simulink model "pendule_simple"  (R2023a)
settings: Solver=VariableStepAuto  StartTime=0.0  StopTime=10.0  RelTol=1e-3
undefined symbols (not defined in the file): g, l
settings Model: Creator=pmt1554  LastModifiedBy=pmt1554

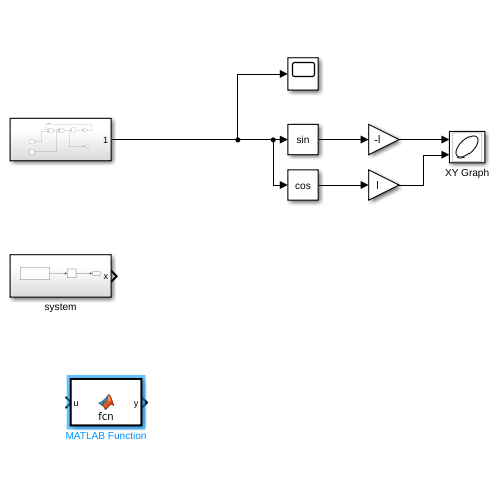
[thumbnail: Simulink's stored preview of the top-level diagram]
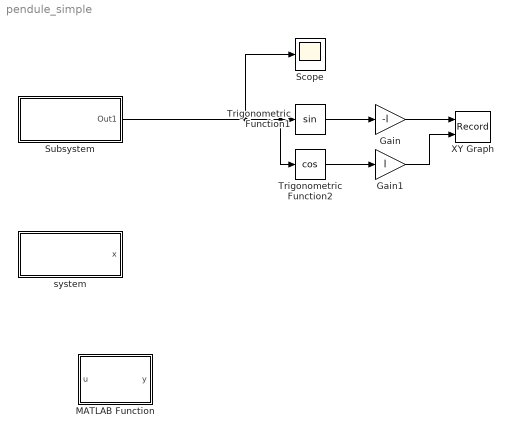
== system pendule_simple ==
  Gain : Gain  Gain=-l
  Gain1 : Gain  Gain=l
  MATLAB Function : MATLAB Function  TreatAsAtomicUnit=on
  Scope : Scope
  Subsystem : Subsystem
  Trigonometric Function1 : Trigonometry
  Trigonometric Function2 : Trigonometry  Operator=cos
  XY Graph : Record  FileSettingsInternal="{\"entries\":[{\"content\":{\"excelSettings\":{\"content\":{},\"type\":\"Streamout.ExcelSettings\"}},\"type\":\"Streamout.FileSettingStorage\",\"uuid\":\"aeae67a6-a75f-4884-904f-e6fdfa875448\"}],\"packageUris\":[\"http://schema.mathworks.com/mf0/streamout_blocks/R2020a\"],\"version\":\"1.0\"}"  Layout=[1 1]  SignalsInternal="{\"entries\":[{\"content\":{\"signals\":[{\"content\":{\"blockPath\":[\"pendule_simple/XY Graph\"],\"dimensions\":[1],\"domain\":\"pendule_simple/XY Graph\",\"lineColor\":\"#a2142f\",\"plots\":[1],\"port\":1,\"sid\":[\"\"],\"signalID\":165,\"signalName\":\"Gain\"},\"type\":\"RecordBlkView.Signal\",\"uuid\":\"293a6cc9-5755-4e67-9070-f33e419323fb\"},{\"content\":{\"blockPath\":[\"pendule_simple/XY Graph\"],\"dimensions\":[1],\"domain\":\"pendule_simple/XY Graph\",\"lineColor\":\"#139fff\",\"plots\":[1],\"port\":2,\"sid\":[\"\"],\"signalID\":169,\"signalName\":\"Gain1\"},\"type\":\"RecordBlkView.Signal\",\"uuid\":\"7e1f4678-e9f9-43f3-9651-46c8d029192f\"}]},\"type\":\"RecordBlkView.InputSignals\",\"uuid\":\"0e4fe57e-2004-49e8-ae38-3160f38942a6\"}],\"packageUris\":[\"http://schema.mathworks.com/mf0/streamout_blocks/R2020a\"],\"version\":\"1.0\"}"  VisualizationBindings="{\"xyplotplugin\":{\"info\":[{\"series\":[{\"bindingParametersList\":[{\"parameter\":\"X-Axis\",\"signalID\":165,\"signalName\":\"Gain\"},{\"parameter\":\"Y-Axis\",\"signalID\":169,\"signalName\":\"Gain1\"}],\"seriesID\":50671}],\"subplotID\":1}]}}"  CompatibilityTag=XY
  system : Subsystem
  wires:
  Subsystem/1(Out1) -> Trigonometric Function2/1, Trigonometric Function1/1, Scope/1
  Trigonometric Function1/1 -> Gain/1
  Gain/1 -> XY Graph/1
  Trigonometric Function2/1 -> Gain1/1
  Gain1/1 -> XY Graph/2

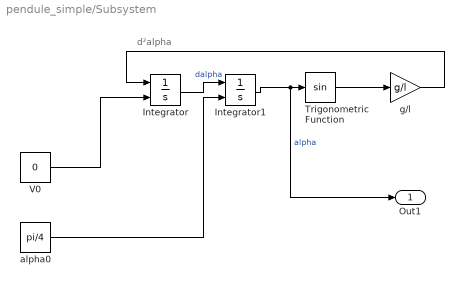
== system pendule_simple/Subsystem ==
  note: d²alpha
  Integrator : Integrator  InitialConditionSource=external  InitialCondition=1
  Integrator1 : Integrator  InitialConditionSource=external  InitialCondition=1
  Trigonometric Function : Trigonometry
  V0 : Constant  Value=0
  alpha0 : Constant  Value=pi/4
  g/l : Gain  Gain=g/l
  Out1 : Outport
  wires:
  V0/1 -> Integrator/2
  Integrator/1 -> Integrator1/1  "dalpha"
  Trigonometric Function/1 -> g/l/1
  Integrator1/1 -> Out1/1, Trigonometric Function/1  "alpha"
  alpha0/1 -> Integrator1/2
  g/l/1 -> Integrator/1

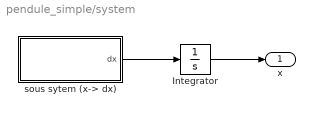
== system pendule_simple/system ==
  Integrator : Integrator
  sous sytem (x-> dx) : Subsystem
  x : Outport
  wires:
  sous sytem (x-> dx)/1(dx) -> Integrator/1
  Integrator/1 -> x/1

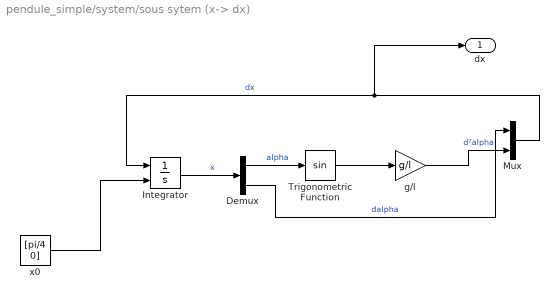
== system pendule_simple/system/sous sytem (x-> dx) ==
  Demux : Demux  Outputs=2
  Integrator : Integrator  InitialConditionSource=external  InitialCondition=1
  Mux : Mux  Inputs=2
  Trigonometric Function : Trigonometry
  g/l : Gain  Gain=g/l
  x0 : Constant  Value=[pi/4 0]
  dx : Outport
  wires:
  Demux/1 -> Trigonometric Function/1  "alpha"
  Mux/1 -> dx/1, Integrator/1  "dx"
  Demux/2 -> Mux/1  "dalpha"
  Trigonometric Function/1 -> g/l/1
  x0/1 -> Integrator/2
  Integrator/1 -> Demux/1  "x"
  g/l/1 -> Mux/2  "d²alpha"

== matlab function pendule_simple/MATLAB Function ==
  data: u input; y output
function y = fcn(u)
    
y = u;
